simulink model "Offline_DataImport_AND_Preprocessing_ECGandSCG3D"  (R2020b)
settings: Solver=FixedStepDiscrete  StartTime=0.0  StopTime=param_sim_time  FixedStep=1/fs  MaxStep=1/fs  RelTol=1e-3
undefined symbols (not defined in the file): fdesignblkfcn, fs, gcbh, param_tot_samples
(part 3 of 3)

== system Offline_DataImport_AND_Preprocessing_ECGandSCG3D/SCG Preprocessing/Enabled SCG Preprocessing Subsystem/Filtfiltering/Bandpass Filter 2 ==
  In : Inport
  Generated Filter Block : DiscreteFir  Tag=BlockMethodSubSystem  Coefficients=[-0.0141280809748904439 0.00296128789229228515 0.00257104999710804256 0.00216178345802768047 0.00175552729414372999 0.00135185618919184472 0.000971465225508600858 0.000611761661220453987 0.000291406420521167497 4.82187739932540826e-06 -0.000231481095028417821 -0.000426883300566277893 -0.000566810793415693445 -0.000665092291782963183 -0.000708283395739488578 -0.000716103852974601593 -0.000671547633475275477 -0.000615106494933681525 -0.000488109909377643092 -0.000390234789954030728 -0.000258144491787600308 -0.000103777427082080848 3.69273719204449291e-05 0.000160217379967343004 0.000266719346682901468 0.000355855181711899407 0.00042444354991033259 0.000465107287062647284 0.000475941357662141781 0.00045436165469465474 0.000405500722307057526 0.000332653752196140906 0.000244041476717768088 0.000145867245103578971 4.31958982817989834e-05 -5.15123314384427489e-05 -0.000142923677775342456 -0.000215518203590111396 -0.000261730266501190856 -0.000295405514048500267 -0.00029258904073516806 -0.000262673662663715293 -0.000200239042161780637 -0.000119059290944066934 -1.21322536877112308e-05 0.000106963831734476281 0.00024029907401433917 0.000369441485674023434 0.000494924114257109735 0.000600074273648323539 0.000689180050721941578 0.000747556211879763649 0.000783700181000823726 0.000783037479294958205 0.000758170640681657751 0.000702221229410942768 0.00062234914182012803 0.000526336913415673471 0.000422160757970439435 0.000311595034642000654 0.000210279303290443823 0.00012116322132581063 5.51843108115603054e-05 1.14901317571792366e-05 4.63268984915096715e-07 1.97600364122418881e-05 7.52585257248264416e-05 0.000158650819102896384 0.000270390241192549133 0.000399318062573107355 0.000542643635713839848 0.000686965575031403888 0.00082909540621049771 0.000950782043587884013 0.00105531510633344837 0.0011243012388455851 0.00116225627563770577 0.00116100403898223951 0.00112659092458904618 0.00105319818945410169 0.000953344560012697739 0.000827179974613592023 0.000689621114973500843 0.000542798204792315636 0.000403935329663590928 0.000276677120819612474 0.000176948147897270508 0.000104790831399949325 7.17507496431589453e-05 7.47958920749892953e-05 0.0001189809160239471 0.000199000478147139462 0.000312036321493172272 0.000446906185270561432 0.000599958367208563298 0.000753866459386062782 0.00090376858726108622 0.00103429112272443793 0.00114049954630186627 0.00120812081357756125 0.00123691779750273109 0.00121863837734643987 0.00115823236504885609 0.00105257319614873897 0.000912433904619841529 0.000740597166721868039 0.000552884553978793408 0.000354055164106317766 0.000163199294344686802 -1.50951637483565798e-05 -0.000162513118388487796 -0.000275080946577539037 -0.000341943188723405761 -0.000363442033376501494 -0.00033415202471282282 -0.000262311282575341045 -0.000148736623332661536 -6.29165138528280099e-06 0.000158313981566005763 0.000327534481367972377 0.000492510275335960451 0.000636058676656042071 0.000750308535347654973 0.000820834153970448691 0.000843500867080383687 0.000811058974000754968 0.000725579145441419826 0.000586861203976211943 0.000405054868711680893 0.000184940546124518629 -5.5900228056928597e-05 -0.000308204861095128652 -0.000553436858002336746 -0.000780717962187617992 -0.000972296884021763008 -0.00112115970011063791 -0.00121428591472381824 -0.00125044236292902976 -0.00122449203339279784 -0.00114390543564522537 -0.00101139494448912459 -0.000841431774385854175 -0.000642541957157717614 -0.000434750691331369996 -0.000229897013949648468 -4.78783601658636093e-05 9.9539490455416782e-05 0.000197094197447343286 0.000237758271413028577 0.00021254671910410014 0.000123930849749381497 -2.84437637916960806e-05 -0.000234134053639612275 -0.000484592671067754152 -0.000762051837015052455 -0.00105285099253676732 -0.00133585896082411525 -0.00159595443115483245 -0.00181366900494322504 -0.00197783075368637359 -0.00207501327682029293 -0.00210124750065167169 -0.00205143676620881017 -0.00193252830137258941 -0.0017485276980914212 -0.00151582984003622266 ...(+13710 chars)]  InputProcessing=Columns as channels (frame based)
  Out : Outport  VectorParamsAs1DForOutWhenUnconnected=off
  wires:
  In/1 -> Generated Filter Block/1
  Generated Filter Block/1 -> Out/1
